simulink model "sfcndemo_matadd"  (R2021a)
settings: Solver=FixedStepDiscrete  StartTime=0.0  StopTime=10.0  RelTol=1e-3
Description:
  | Matrix-Add (Bias) Using One Input and One Parameter C-MEX S-function
settings Model: ExtModeAutoUpdateStatusClock=off  Creator=The MathWorks, Inc.  LastModifiedBy=landon
settings SolverCC: AlgebraicLoopSolver=TrustRegion
settings DataIOCC: LimitDataPoints=on  SaveFormat=Array  SaveOutput=off  OutputSaveName=y1,y2,y3,y4
settings OptimizationCC: BlockReduction=off  BooleanDataType=off  ExpressionDepthLimit=2147483647  InitFltsAndDblsToZero=on  LifeSpan=inf
settings DebuggingCC: SaveWithParameterizedLinksMsg=none  SignalResolutionControl=TryResolveAllWithWarning  MultiTaskDSMMsg=warning  MultiTaskCondExecSysMsg=none  FcnCallInpInsideContextMsg=warning  StateNameClashWarn=warning  SFUnexpectedBacktrackingDiag=warning  SFNoUnconditionalDefaultTransitionDiag=warning  SFExecutionAtInitializationDiag=none  SFMachineParentedDataDiag=warning  ArithmeticOperatorsInVariantConditions=warning
settings HardwareCC: ProdBitPerPointer=32  ProdBitPerSizeT=32  ProdBitPerPtrDiffT=32  ProdLargestAtomicFloat=None  ProdIntDivRoundTo=Undefined  ProdEndianess=Unspecified  ProdWordSize=32  ProdHWDeviceType=32-bit Generic  TargetBitPerLong=64  TargetBitPerPointer=64  TargetBitPerSizeT=64  TargetBitPerPtrDiffT=64  TargetLongLongMode=on  TargetIntDivRoundTo=Zero  TargetEndianess=LittleEndian  TargetWordSize=64  TargetHWDeviceType=MATLAB Host  ProdEqTarget=off
settings ModelReferenceCC: PropagateSignalLabelsOutOfModel=off
settings SFSimCC: SimUseLocalCustomCode=off  CustomCodeUndefinedFunction=UseInterfaceOnly
settings RTWCC: GenCodeOnly=on  PackageGeneratedCodeAndArtifacts=on  RTWUseLocalCustomCode=off
settings CodeAppCC: StateflowObjectComments=on
settings GRTTargetCC: TargetFcnLib=ansi_tfl_tmw.mat  TargetLangStandard=C89/C90 (ANSI)  RTWCAPISignals=on  RTWCAPIParams=on  RTWCAPIStates=on  RTWCAPIRootIO=on
settings ConfigComp: CovMetricSettings=dw  CovSaveCumulativeToWorkspaceVar=on  CovSaveSingleToWorkspaceVar=on  CovExternalEMLEnable=off

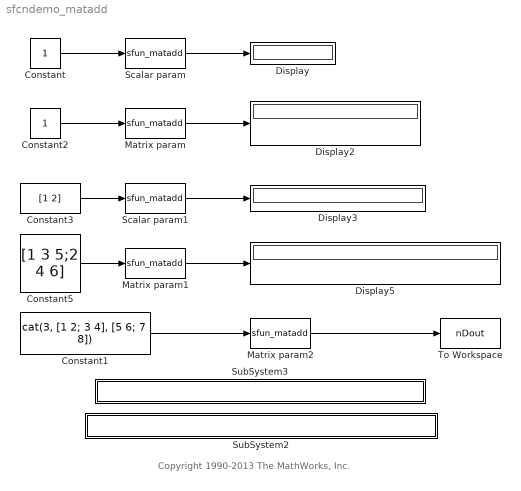
== system sfcndemo_matadd ==
  note: Copyright 1990-2013 The MathWorks, Inc.
  Constant : Constant  VectorParams1D=off
  Constant1 : Constant  Value=cat(3, [1 2; 3 4], [5 6; 7 8])  VectorParams1D=off
  Constant2 : Constant  VectorParams1D=off
  Constant3 : Constant  Value=[1 2]  VectorParams1D=off
  Constant5 : Constant  Value=[1 3 5;2 4 6]  VectorParams1D=off
  Display{,2..3,5} (4 alike) : Display
  Matrix param : S-Function  FunctionName=sfun_matadd  Parameters=Operand  SFunctionDeploymentMode=off  EnableBusSupport=off  mask(Matrix add){Operand=[1 3; 2 4]}
      mask prompts: Operand "Operand 1:"
      settings: AttributesFormatString=Param = %<Operand>
      mask Display: disp('Matrix\n Add ')
  Matrix param1 : S-Function  FunctionName=sfun_matadd  Parameters=Operand  SFunctionDeploymentMode=off  EnableBusSupport=off  mask(Matrix add){Operand=[1 3 5;2 4 6]}
      mask prompts: Operand "Operand 1:"
      settings: AttributesFormatString=Param = %<Operand>
      mask Display: disp('Matrix\n Add ')
  Matrix param2 : S-Function  FunctionName=sfun_matadd  Parameters=Operand  SFunctionDeploymentMode=off  EnableBusSupport=off  mask(Matrix add){Operand=cat(3, [1 2; 3 4], [5 6; 7 8])}
      mask prompts: Operand "Operand 1:"
      settings: AttributesFormatString=Param = %<Operand>
      mask Display: disp('Matrix\n Add ')
  Scalar param : S-Function  FunctionName=sfun_matadd  Parameters=Operand  SFunctionDeploymentMode=off  EnableBusSupport=off  mask(Matrix add){Operand=1}
      mask prompts: Operand "Operand 1:"
      settings: AttributesFormatString=Param = %<Operand>
      mask Display: disp('Matrix\n Add ')
  Scalar param1 : S-Function  FunctionName=sfun_matadd  Parameters=Operand  SFunctionDeploymentMode=off  EnableBusSupport=off  mask(Matrix add){Operand=1}
      mask prompts: Operand "Operand 1:"
      settings: AttributesFormatString=Param = %<Operand>
      mask Display: disp('Matrix\n Add ')
  SubSystem2 : Subsystem  mask{filename=sfun_matadd.tlc}
      mask init:
      | x=sfundemo_maskdisp;
      settings: AttributesFormatString=\n  OpenFcn=sfundemo_openfcn
      mask Display: disp(x);
  SubSystem3 : Subsystem  mask{filename=sfun_matadd.c}
      mask init:
      | x=sfundemo_maskdisp;
      settings: AttributesFormatString=\n  OpenFcn=sfundemo_openfcn
      mask Display: disp(x);
  To Workspace : ToWorkspace  VariableName=nDout  SaveFormat=Structure  SampleTime=-1
  wires:
  Constant/1 -> Scalar param/1
  Scalar param/1 -> Display/1
  Constant2/1 -> Matrix param/1
  Matrix param/1 -> Display2/1
  Constant3/1 -> Scalar param1/1
  Scalar param1/1 -> Display3/1
  Constant5/1 -> Matrix param1/1
  Matrix param1/1 -> Display5/1
  Constant1/1 -> Matrix param2/1
  Matrix param2/1 -> To Workspace/1

== system sfcndemo_matadd/SubSystem2 ==

== system sfcndemo_matadd/SubSystem3 ==
